simulink model "sampleModel1424"  (R2023a)
settings: Solver=VariableStepAuto  StartTime=0.0  StopTime=10.0  RelTol=1e-3
libraries: hdlsllib x2, simulink x1
settings Model: Creator=user1  LastModifiedBy=user1

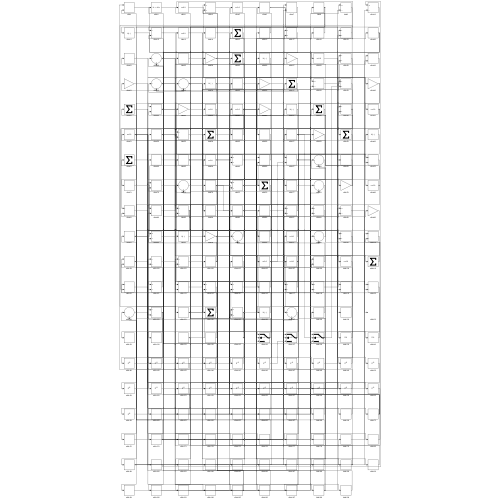
[thumbnail: Simulink's stored preview of the top-level diagram]
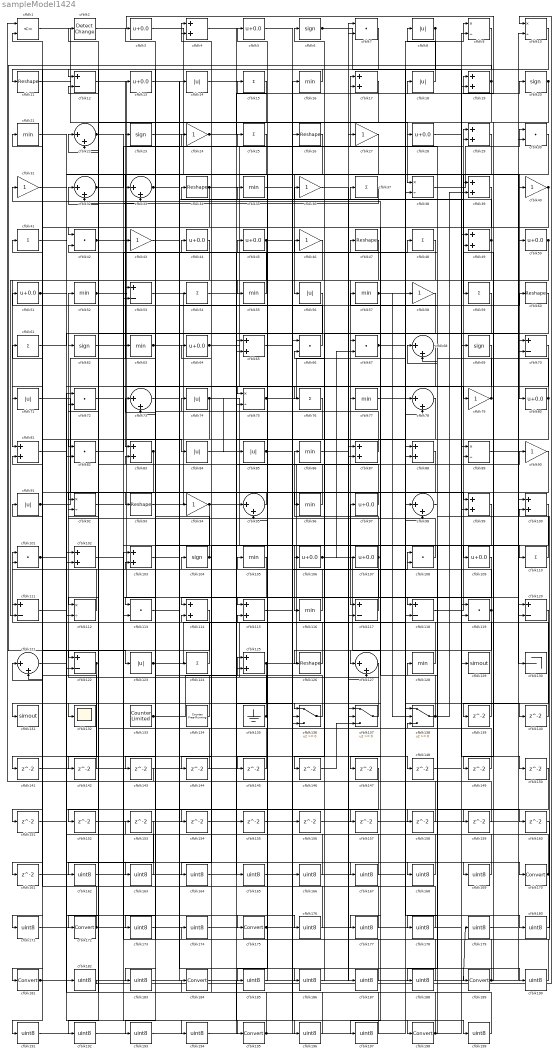
== system sampleModel1424 ==
  cfblk1 : RelationalOperator  Operator=<=  OutDataTypeStr=boolean  InputSameDT=off
  cfblk{9..10,38,75,89,92,112} (7 alike) : Product  Inputs=*/  RndMeth=Zero  SaturateOnIntegerOverflow=on
  cfblk{4,17,19,29,39,49,65,81,83,87..88,99..100,102..103,114..115,125} (18 alike) : Sum
  cfblk{7,30,42,66..67,72,82,101,108,113,119} (11 alike) : DotProduct  OutDataTypeStr=Inherit: Inherit via internal rule
  cfblk{6,20,23,62,69,104} (6 alike) : Signum
  cfblk{16,21,35,52,55,57,63,77,86,96,105,116,128} (13 alike) : MinMax
  cfblk{3,5,13,28,44..45,50..51,64,80,97,106..107,109} (14 alike) : Bias  Bias=0.0  SaturateOnIntegerOverflow=off
  cfblk{11,26,34,47,60,93,126} (7 alike) : Reshape
  cfblk{15,25,37,41,48,54,59,61,76,110,124} (11 alike) : Sum  Inputs=+
  cfblk{12,53,70,111,117..118,120,122} (8 alike) : Sum  Inputs=+-
  cfblk{22,32..33,68,73,78,95,98,121,127} (10 alike) : Sum  Inputs=|++
  cfblk{8,14,18,56,71,74,84..85,91,123} (10 alike) : Abs  SaturateOnIntegerOverflow=off
  cfblk129 : ToWorkspace  VariableName=simout  SaveFormat=Timeseries  SampleTime=-1
  cfblk130 : Terminator
  cfblk131 : ToWorkspace  VariableName=simout  SaveFormat=Timeseries  SampleTime=-1
  cfblk132 : Scope
  cfblk133 : hdlsllib/Sources/Counter Limited  uplimit=7  tsamp=-1
  cfblk134 : hdlsllib/Sources/Counter Free-Running  NumBits=16  tsamp=-1
  cfblk135 : Ground
  cfblk136 : Switch  SaturateOnIntegerOverflow=off  InputSameDT=off
  cfblk137 : Switch  SaturateOnIntegerOverflow=off  InputSameDT=off
  cfblk138 : Switch  SaturateOnIntegerOverflow=off  InputSameDT=off
  cfblk{139..161} (23 alike) : Delay  SampleTime=1
  cfblk{162..169,171,173..174,176..180,182..183,185..188,190..194,196..197,199} (30 alike) : DataTypeConversion  OutDataTypeStr=uint8  SaturateOnIntegerOverflow=off  RndMeth=Floor
  cfblk{170,172,175,181,184,189,195,198} (8 alike) : DataTypeConversion  SaturateOnIntegerOverflow=off  RndMeth=Floor
  cfblk2 : simulink/Logic and Bit Operations/Detect Change  vinit=0  OutDataTypeStr=boolean
      settings: LibrarySourceBlock=|
      | hdlsllib/Logic and Bit
      | Operations/Detect
      | Change
  cfblk{24,27,31,36,40,43,46,58,79,90,94} (11 alike) : Gain
  wires:
  cfblk125/1 -> cfblk90/1, cfblk154/1
  cfblk12/1 -> cfblk115/1
  cfblk50/1 -> cfblk53/1, cfblk145/1
  cfblk118/1 -> cfblk29/1
  cfblk127/1 -> cfblk25/1
  cfblk47/1 -> cfblk81/1
  cfblk87/1 -> cfblk51/1
  cfblk106/1 -> cfblk132/1, cfblk67/2
  cfblk108/1 -> cfblk52/1
  cfblk26/1 -> cfblk56/1
  cfblk133/1 -> cfblk125/1, cfblk183/1
  cfblk53/1 -> cfblk99/1
  cfblk29/1 -> cfblk59/1
  cfblk19/1 -> cfblk123/1, cfblk42/1
  cfblk64/1 -> cfblk17/1, cfblk127/2
  cfblk11/1 -> cfblk138/1
  cfblk23/1 -> cfblk80/1
  cfblk137/1 -> cfblk62/1
  cfblk49/1 -> cfblk117/1, cfblk53/2, cfblk4/1
  cfblk107/1 -> cfblk86/1, cfblk185/1
  cfblk138/1 -> cfblk31/1, cfblk39/2
  cfblk7/1 -> cfblk172/1
  cfblk20/1 -> cfblk28/1, cfblk136/2, cfblk149/1
  cfblk80/1 -> cfblk44/1, cfblk146/1
  cfblk66/1 -> cfblk21/1
  cfblk51/1 -> cfblk96/1, cfblk159/1, cfblk160/1
  cfblk63/1 -> cfblk79/1, cfblk60/1
  cfblk74/1 -> cfblk116/1, cfblk85/1, cfblk88/2, cfblk151/1
  cfblk79/1 -> cfblk57/1, cfblk23/1
  cfblk24/1 -> cfblk17/2, cfblk136/3
  cfblk117/1 -> cfblk97/1
  cfblk122/1 -> cfblk131/1, cfblk171/1
  cfblk45/1 -> cfblk122/2, cfblk18/1, cfblk87/2, cfblk190/1
  cfblk121/1 -> cfblk175/1
  cfblk32/1 -> cfblk29/2, cfblk176/1
  cfblk54/1 -> cfblk170/1
  cfblk1/1 -> cfblk38/1
  cfblk112/1 -> cfblk61/1
  cfblk91/1 -> cfblk13/1, cfblk148/1
  cfblk37/1 -> cfblk32/2
  cfblk71/1 -> cfblk93/1
  cfblk85/1 -> cfblk16/1, cfblk20/1
  cfblk2/1 -> cfblk19/1
  cfblk8/1 -> cfblk113/1, cfblk73/2
  cfblk89/1 -> cfblk130/1
  cfblk115/1 -> cfblk108/1
  cfblk21/1 -> cfblk40/1
  cfblk43/1 -> cfblk37/1
  cfblk109/1 -> cfblk114/1
  cfblk77/1 -> cfblk110/1
  cfblk101/1 -> cfblk41/1, cfblk163/1
  cfblk46/1 -> cfblk112/1
  cfblk126/1 -> cfblk114/2
  cfblk42/1 -> cfblk84/1, cfblk12/2, cfblk106/1
  cfblk59/1 -> cfblk136/1
  cfblk62/1 -> cfblk119/1
  cfblk61/1 -> cfblk70/1
  cfblk123/1 -> cfblk98/2, cfblk39/1
  cfblk38/1 -> cfblk30/1
  cfblk3/1 -> cfblk120/1
  cfblk33/1 -> cfblk77/1, cfblk158/1
  cfblk128/1 -> cfblk101/1
  cfblk75/1 -> cfblk9/1, cfblk107/1
  cfblk6/1 -> cfblk69/1, cfblk58/1
  cfblk14/1 -> cfblk109/1
  cfblk83/1 -> cfblk141/1, cfblk191/1
  cfblk65/1 -> cfblk189/1
  cfblk27/1 -> cfblk83/1
  cfblk97/1 -> cfblk22/2
  cfblk34/1 -> cfblk43/1, cfblk157/1
  cfblk98/1 -> cfblk68/2
  cfblk113/1 -> cfblk118/1
  cfblk82/1 -> cfblk47/1
  cfblk56/1 -> cfblk82/1
  cfblk13/1 -> cfblk124/1
  cfblk119/1 -> cfblk95/2, cfblk126/1
  cfblk67/1 -> cfblk70/2, cfblk140/1
  cfblk40/1 -> cfblk50/1, cfblk127/1
  cfblk55/1 -> cfblk2/1
  cfblk102/1 -> cfblk120/2
  cfblk9/1 -> cfblk12/1
  cfblk15/1 -> cfblk122/1
  cfblk10/1 -> cfblk181/1
  cfblk95/1 -> cfblk92/1
  cfblk18/1 -> cfblk8/1
  cfblk68/1 -> cfblk75/1
  cfblk69/1 -> cfblk137/2
  cfblk116/1 -> cfblk91/1
  cfblk134/1 -> cfblk33/1
  cfblk136/1 -> cfblk3/1
  cfblk96/1 -> cfblk83/2
  cfblk70/1 -> cfblk113/2
  cfblk72/1 -> cfblk195/1
  cfblk110/1 -> cfblk46/1
  cfblk30/1 -> cfblk55/1
  cfblk16/1 -> cfblk11/1
  cfblk22/1 -> cfblk33/2, cfblk169/1
  cfblk124/1 -> cfblk111/1
  cfblk31/1 -> cfblk76/1
  cfblk73/1 -> cfblk14/1
  cfblk94/1 -> cfblk48/1, cfblk89/2, cfblk173/1
  cfblk25/1 -> cfblk112/2
  cfblk57/1 -> cfblk118/2, cfblk138/2, cfblk180/1
  cfblk44/1 -> cfblk111/2
  cfblk93/1 -> cfblk99/2
  cfblk135/1 -> cfblk45/1, cfblk73/1
  cfblk90/1 -> cfblk102/2
  cfblk52/1 -> cfblk67/1, cfblk129/1
  cfblk104/1 -> cfblk63/1, cfblk74/1
  cfblk39/1 -> cfblk71/1
  cfblk120/1 -> cfblk139/1
  cfblk139/1 -> cfblk68/1
  cfblk140/1 -> cfblk115/2
  cfblk141/1 -> cfblk95/1
  cfblk17/1 -> cfblk142/1
  cfblk142/1 -> cfblk81/2
  cfblk76/1 -> cfblk143/1
  cfblk143/1 -> cfblk1/1
  cfblk99/1 -> cfblk144/1
  cfblk144/1 -> cfblk92/2
  cfblk145/1 -> cfblk22/1
  cfblk146/1 -> cfblk137/3
  cfblk60/1 -> cfblk147/1
  cfblk148/1 -> cfblk119/2
  cfblk149/1 -> cfblk32/1
  cfblk28/1 -> cfblk150/1
  cfblk151/1 -> cfblk82/2
  cfblk88/1 -> cfblk152/1
  cfblk152/1 -> cfblk49/1
  cfblk154/1 -> cfblk75/2
  cfblk4/1 -> cfblk155/1
  cfblk155/1 -> cfblk117/2
  cfblk156/1 -> cfblk30/2
  cfblk157/1 -> cfblk19/2
  cfblk158/1 -> cfblk1/2
  cfblk159/1 -> cfblk137/1
  cfblk114/1 -> cfblk161/1
  cfblk161/1 -> cfblk98/1
  cfblk153/1 -> cfblk162/1
  cfblk162/1 -> cfblk38/2
  cfblk163/1 -> cfblk153/1
  cfblk105/1 -> cfblk164/1
  cfblk164/1 -> cfblk125/2
  cfblk84/1 -> cfblk165/1
  cfblk165/1 -> cfblk105/1
  cfblk35/1 -> cfblk166/1
  cfblk166/1 -> cfblk102/1
  cfblk111/1 -> cfblk167/1
  cfblk167/1 -> cfblk35/1
  cfblk36/1 -> cfblk168/1
  cfblk168/1 -> cfblk34/1
  cfblk169/1 -> cfblk36/1
  cfblk170/1 -> cfblk4/2, cfblk66/2, cfblk42/2, cfblk128/1
  cfblk171/1 -> cfblk54/1
  cfblk172/1 -> cfblk87/1, cfblk88/1, cfblk101/2, cfblk89/1
  cfblk173/1 -> cfblk7/1
  cfblk160/1 -> cfblk174/1
  cfblk174/1 -> cfblk7/2
  cfblk175/1 -> cfblk156/1, cfblk15/1
  cfblk176/1 -> cfblk121/1
  cfblk58/1 -> cfblk177/1
  cfblk177/1 -> cfblk121/2
  cfblk100/1 -> cfblk178/1
  cfblk178/1 -> cfblk66/1
  cfblk179/1 -> cfblk100/1
  cfblk180/1 -> cfblk100/2
  cfblk181/1 -> cfblk179/1, cfblk94/1, cfblk27/1
  cfblk81/1 -> cfblk182/1
  cfblk182/1 -> cfblk10/1
  cfblk183/1 -> cfblk10/2
  cfblk184/1 -> cfblk198/1
  cfblk185/1 -> cfblk5/1
  cfblk103/1 -> cfblk186/1
  cfblk186/1 -> cfblk6/1
  cfblk86/1 -> cfblk187/1
  cfblk187/1 -> cfblk103/1
  cfblk150/1 -> cfblk188/1
  cfblk188/1 -> cfblk103/2
  cfblk189/1 -> cfblk138/3, cfblk49/2
  cfblk190/1 -> cfblk65/1
  cfblk191/1 -> cfblk65/2
  cfblk78/1 -> cfblk192/1
  cfblk192/1 -> cfblk26/1
  cfblk147/1 -> cfblk193/1
  cfblk193/1 -> cfblk78/1
  cfblk92/1 -> cfblk194/1
  cfblk194/1 -> cfblk78/2
  cfblk195/1 -> cfblk104/1, cfblk64/1
  cfblk41/1 -> cfblk196/1
  cfblk196/1 -> cfblk72/1
  cfblk48/1 -> cfblk197/1
  cfblk197/1 -> cfblk72/2
  cfblk198/1 -> cfblk9/2, cfblk108/2, cfblk24/1
  cfblk5/1 -> cfblk199/1
  cfblk199/1 -> cfblk184/1
